simulink model "ben3bsys"  (Simulink 6.0)
settings: Solver=ode45  SolverMode=SingleTasking  StartTime=0.0  StopTime=4  RelTol=1e-3  AbsTol=1e-6
PreLoadFcn:
  | ben3bdat
values from neighbouring files (symbols this model uses):
  gd1 = 1    [ben2adat.m]    (also in ben3adat.m = [1,6,13])
  gd12 = [1/325/325,0.5/325,1]    [ben2adat.m]
  gd3 = [1/85/85,1.2/85,1]    [ben2adat.m]    (also in ben3adat.m = [1,-1])
  gd4 = 1    [ben2adat.m]    (also in ben3adat.m = [1,-0.6667])
  gd5 = [1/170,1]    [ben2adat.m]    (also in ben3adat.m = [1,-1])
  gd6 = [1,-0.6873]    [ben3adat.m]
  gd7 = [1,0]    [ben2adat.m]    (also in ben3adat.m = [1,-0.9277])
  gd91 = [1,0]    [ben2adat.m]
  gd92 = [1/50,1]    [ben2adat.m]
  gn12 = [1,0]    [ben2adat.m]
  gn1_gn2 = [gn1; gn2]    [ben3adat.m]
  gn3 = 1    [ben2adat.m]    (also in ben3adat.m = .2625*[1,-0.9048])
  gn4 = 1    [ben2adat.m]    (also in ben3adat.m = 1.7*[1,-0.9608])
  gn5 = 1    [ben2adat.m]    (also in ben3adat.m = 1.035*[1,-0.9324])
  gn6 = 0.1564*[1,1]    [ben3adat.m]
  gn7 = 1    [ben2adat.m]    (also in ben3adat.m = 0.0362*[1,1])
  gn91 = [1,1.5]    [ben2adat.m]
  gn92 = [1/150,1]    [ben2adat.m]
  offT1 = 0.0    (= 0)    [ben3adat.m]
  offT2 = 0.00499999    [ben3adat.m]
  offZOH = 1.0e-8    (= 1e-08)    [ben3adat.m]
  T1 = 1/50    (= 0.02)    [ben3adat.m]
  T2 = 1/200    (= 0.005)    [ben3adat.m]
undefined symbols (not defined in the file or in its folder): gd101, gd102, gd111, gd112, gd113, gd131, gd132, gd81, gd82, gn101, gn102, gn111, gn112, gn113, gn131, gn132, gn81, gn82, offT3, offT4, T3, T4
settings Model: Creator=The MathWorks Inc.  LastModifiedBy=batserve  ExtModeTrigMode=oneshot  ExtModeArmWhenConnect=off  ExtModeAutoUpdateStatusClock=off
settings DataIOCC: ExternalInput=[]  InitialState=[]  LimitDataPoints=off  SaveOutput=off  SaveTime=off
settings OptimizationCC: BooleanDataType=off
settings DebuggingCC: CheckExecutionContextPreStartOutputMsg=on  CheckExecutionContextRuntimeOutputMsg=on  SolverPrmCheckMsg=none  IntegerOverflowMsg=none
settings HardwareCC: TargetUnknown=on

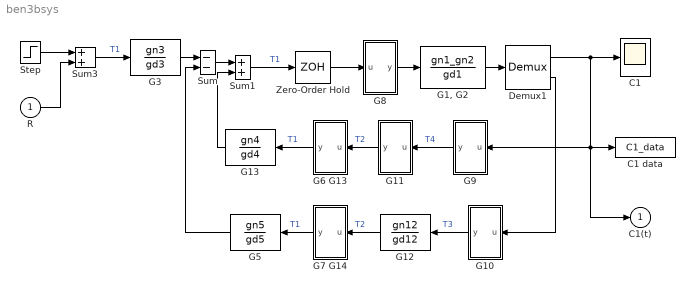
== system ben3bsys ==
  R : Inport  Port=1  LatchInput=off
  C1 : Scope
      settings: TickLabels=on  YMin=0  YMax=1.5  DataFormat=Array
  C1 data : ToWorkspace  VariableName=C1_data  SampleTime=-1  SaveFormat=Array
      settings: MaxDataPoints=20000
  Demux1 : Demux  Outputs=2
  "G1, G2" : TransferFcn  Numerator=gn1_gn2  Denominator=gd1
  G10 : Subsystem  Orientation=left  PropExecContextAcrossSSBoundary=on
  G11 : Subsystem  Orientation=left  PropExecContextAcrossSSBoundary=on
  G12 : DiscreteTransferFcn  Orientation=left  Numerator=gn12  Denominator=gd12  SampleTime=[T3,offT3]
  G13 : DiscreteTransferFcn  Orientation=left  Numerator=gn4  Denominator=gd4  SampleTime=[T1,offT1]
  G3 : DiscreteTransferFcn  Numerator=gn3  Denominator=gd3  SampleTime=[T1,offT1]
  G5 : DiscreteTransferFcn  Orientation=left  Numerator=gn5  Denominator=gd5  SampleTime=[T1,offT1]
  G6 G13 : Subsystem  Orientation=left  PropExecContextAcrossSSBoundary=on
  G7 G14 : Subsystem  Orientation=left  PropExecContextAcrossSSBoundary=on
  G8 : Subsystem  PropExecContextAcrossSSBoundary=on
  G9 : Subsystem  Orientation=left  PropExecContextAcrossSSBoundary=on
  Step : Step  Time=0  SampleTime=0
  Sum : Sum  Inputs=--  SaturateOnIntegerOverflow=on  InputSameDT=on
  Sum1 : Sum  Inputs=2  SaturateOnIntegerOverflow=on  InputSameDT=on
  Sum3 : Sum  SaturateOnIntegerOverflow=on  InputSameDT=on
  Zero-Order Hold : ZeroOrderHold  SampleTime=[T1,offZOH]
  C1(t) : Outport  InitialOutput=0
  wires:
  G5/1 -> Sum/2
  G7 G14/1(y) -> G5/1  "T1"
  G12/1 -> G7 G14/1(u)  "T2"
  G10/1(y) -> G12/1  "T3"
  G6 G13/1(y) -> G13/1  "T1"
  G11/1(y) -> G6 G13/1(u)  "T2"
  G9/1(y) -> G11/1(u)  "T4"
  Zero-Order Hold/1 -> G8/1(u)
  Sum1/1 -> Zero-Order Hold/1  "T1"
  G13/1 -> Sum1/2
  Sum/1 -> Sum1/1
  G3/1 -> Sum/1
  Sum3/1 -> G3/1  "T1"
  G8/1(y) -> "G1, G2"/1
  "G1, G2"/1 -> Demux1/1
  Demux1/1 -> C1/1, C1 data/1, G9/1(u), C1(t)/1
  Demux1/2 -> G10/1(u)
  Step/1 -> Sum3/1
  R/1 -> Sum3/2

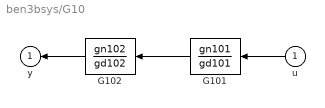
== system ben3bsys/G10 ==
  u : Inport  Orientation=left  Port=1  LatchInput=off
  G101 : TransferFcn  Orientation=left  Numerator=gn101  Denominator=gd101
  G102 : TransferFcn  Orientation=left  Numerator=gn102  Denominator=gd102
  y : Outport  Orientation=left  InitialOutput=0
  wires:
  G102/1 -> y/1
  G101/1 -> G102/1
  u/1 -> G101/1

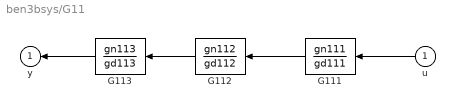
== system ben3bsys/G11 ==
  u : Inport  Orientation=left  Port=1  LatchInput=off
  G111 : DiscreteTransferFcn  Orientation=left  Numerator=gn111  Denominator=gd111  SampleTime=[T4,offT4]
  G112 : DiscreteTransferFcn  Orientation=left  Numerator=gn112  Denominator=gd112  SampleTime=[T4,offT4]
  G113 : DiscreteTransferFcn  Orientation=left  Numerator=gn113  Denominator=gd113  SampleTime=[T4,offT4]
  y : Outport  Orientation=left  InitialOutput=0
  wires:
  u/1 -> G111/1
  G111/1 -> G112/1
  G112/1 -> G113/1
  G113/1 -> y/1

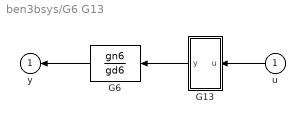
== system ben3bsys/G6 G13 ==
  u : Inport  Orientation=left  Port=1  LatchInput=off
  G13 : Subsystem  Orientation=left  PropExecContextAcrossSSBoundary=on
  G6 : DiscreteTransferFcn  Orientation=left  Numerator=gn6  Denominator=gd6  SampleTime=[T2,offT2]
  y : Outport  Orientation=left  InitialOutput=0
  wires:
  u/1 -> G13/1(u)
  G6/1 -> y/1
  G13/1(y) -> G6/1

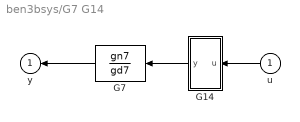
== system ben3bsys/G7 G14 ==
  u : Inport  Orientation=left  Port=1  LatchInput=off
  G14 : Subsystem  Orientation=left  PropExecContextAcrossSSBoundary=on
  G7 : DiscreteTransferFcn  Orientation=left  Numerator=gn7  Denominator=gd7  SampleTime=[T2,offT2]
  y : Outport  Orientation=left  InitialOutput=0
  wires:
  G7/1 -> y/1
  u/1 -> G14/1(u)
  G14/1(y) -> G7/1

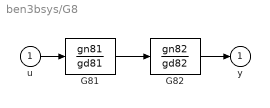
== system ben3bsys/G8 ==
  u : Inport  Port=1  LatchInput=off
  G81 : TransferFcn  Numerator=gn81  Denominator=gd81
  G82 : TransferFcn  Numerator=gn82  Denominator=gd82
  y : Outport  InitialOutput=0
  wires:
  G82/1 -> y/1
  G81/1 -> G82/1
  u/1 -> G81/1

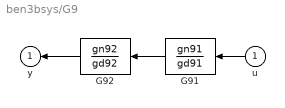
== system ben3bsys/G9 ==
  u : Inport  Orientation=left  Port=1  LatchInput=off
  G91 : TransferFcn  Orientation=left  Numerator=gn91  Denominator=gd91
  G92 : TransferFcn  Orientation=left  Numerator=gn92  Denominator=gd92
  y : Outport  Orientation=left  InitialOutput=0
  wires:
  u/1 -> G91/1
  G91/1 -> G92/1
  G92/1 -> y/1

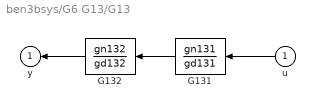
== system ben3bsys/G6 G13/G13 ==
  u : Inport  Orientation=left  Port=1  LatchInput=off
  G131 : DiscreteTransferFcn  Orientation=left  Numerator=gn131  Denominator=gd131  SampleTime=[T2,offT2]
  G132 : DiscreteTransferFcn  Orientation=left  Numerator=gn132  Denominator=gd132  SampleTime=[T2,offT2]
  y : Outport  Orientation=left  InitialOutput=0
  wires:
  u/1 -> G131/1
  G131/1 -> G132/1
  G132/1 -> y/1

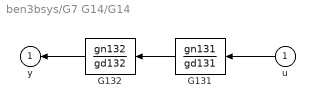
== system ben3bsys/G7 G14/G14 ==
  u : Inport  Orientation=left  Port=1  LatchInput=off
  G131 : DiscreteTransferFcn  Orientation=left  Numerator=gn131  Denominator=gd131  SampleTime=[T2,offT2]
  G132 : DiscreteTransferFcn  Orientation=left  Numerator=gn132  Denominator=gd132  SampleTime=[T2,offT2]
  y : Outport  Orientation=left  InitialOutput=0
  wires:
  u/1 -> G131/1
  G131/1 -> G132/1
  G132/1 -> y/1
